simulink model "IEEE34BARRAS"  (R2018a)
settings: Solver=ode4  StartTime=0.0  StopTime=48*T  FixedStep=Ts  RelTol=1e-3  EnableMultiTasking=on
InitFcn:
  | close
  | clc
  | clear
  | n=2^8;
  | f=60;
  | T=1/f;
  | Ts=1/(f*n);
  | NT=18;
  | set_param('IEEE34BARRAS/EMISOR-RECEPTOR/TCP_IP_RX1/ESCRITURA', 'Value','[0,0,0,0,0,0,0,0,0,0,0,0,0,0,0,0,0,0,0,0,0,0,0,0,0,0,0,0,0,0,0,0,0,0,0,0,0,0,0,0,0]')
  | set_param('IEEE34BARRAS/EMISOR-RECEPTOR/TCP_IP_RX1/RETARDO', 'Value','0')
  | run script_client_1_inicio1.m
undefined symbols (not defined in the file or in its folder): D1, Delta, DiscIntNeverNeededParam, Ip1
libraries: powerlib x313, simulink x15, libreria_medidores1 x3, libreria_comunicaciones_cliente1 x2
(part 3 of 5)

== system IEEE34BARRAS/836-862 ==
  Ground : powerlib/Elements/Ground  LConnTagsString=a
  Series RLC Branch1 : powerlib/Elements/Series RLC Branch  LConnTagsString=__new0  RConnTagsString=__new0  BranchType=RL  Resistance=R(1)*Ft  Inductance=L(1)*Ft  SetiL0=off  InitialCurrent=0  Capacitance=8.4659e-09  Setx0=off  InitialVoltage=0  Measurements=None
  Series RLC Branch11 : powerlib/Elements/Series RLC Branch  LConnTagsString=__new0  RConnTagsString=__new0  BranchType=C  Resistance=0.13252  Inductance=0.0024863  SetiL0=off  InitialCurrent=0  Capacitance=C(1)/2*Ft  Setx0=off  InitialVoltage=0  Measurements=None
  Series RLC Branch12 : powerlib/Elements/Series RLC Branch  LConnTagsString=__new0  RConnTagsString=__new0  BranchType=C  Resistance=0.13252  Inductance=0.0024863  SetiL0=off  InitialCurrent=0  Capacitance=C(3)/2*Ft  Setx0=off  InitialVoltage=0  Measurements=None
  Series RLC Branch13 : powerlib/Elements/Series RLC Branch  LConnTagsString=__new0  RConnTagsString=__new0  BranchType=C  Resistance=0.13252  Inductance=0.0024863  SetiL0=off  InitialCurrent=0  Capacitance=C(3)/2*Ft  Setx0=off  InitialVoltage=0  Measurements=None
  Series RLC Branch2 : powerlib/Elements/Series RLC Branch  LConnTagsString=__new0  RConnTagsString=__new0  BranchType=RL  Resistance=R(2)*Ft  Inductance=L(2)*Ft  SetiL0=off  InitialCurrent=0  Capacitance=8.4659e-09  Setx0=off  InitialVoltage=0  Measurements=None
  Series RLC Branch3 : powerlib/Elements/Series RLC Branch  LConnTagsString=__new0  RConnTagsString=__new0  BranchType=C  Resistance=0.13252  Inductance=0.0024863  SetiL0=off  InitialCurrent=0  Capacitance=C(2)/2*Ft  Setx0=off  InitialVoltage=0  Measurements=None
  Series RLC Branch7 : powerlib/Elements/Series RLC Branch  LConnTagsString=__new0  RConnTagsString=__new0  BranchType=C  Resistance=0.13252  Inductance=0.0024863  SetiL0=off  InitialCurrent=0  Capacitance=C(1)/2*Ft  Setx0=off  InitialVoltage=0  Measurements=None
  Series RLC Branch8 : powerlib/Elements/Series RLC Branch  LConnTagsString=__new0  RConnTagsString=__new0  BranchType=C  Resistance=0.13252  Inductance=0.0024863  SetiL0=off  InitialCurrent=0  Capacitance=C(2)/2*Ft  Setx0=off  InitialVoltage=0  Measurements=None
  Series RLC Branch9 : powerlib/Elements/Series RLC Branch  LConnTagsString=__new0  RConnTagsString=__new0  BranchType=RL  Resistance=R(3)*Ft  Inductance=L(3)*Ft  SetiL0=off  InitialCurrent=0  Capacitance=8.4659e-09  Setx0=off  InitialVoltage=0  Measurements=None
  B : PMIOPort  Side=Left
  b : PMIOPort  Port=2  Side=Right
  A : PMIOPort  Port=3  Side=Left
  a : PMIOPort  Port=4  Side=Right
  C : PMIOPort  Port=5  Side=Left
  c : PMIOPort  Port=6  Side=Right
  connections:
  B/RConn1 -- Series RLC Branch11/LConn1 -- Series RLC Branch1/LConn1
  b/RConn1 -- Series RLC Branch7/LConn1 -- Series RLC Branch1/RConn1
  Series RLC Branch8/RConn1 -- Series RLC Branch11/RConn1 -- Series RLC Branch13/RConn1 -- Series RLC Branch12/RConn1 -- Series RLC Branch3/RConn1 -- Series RLC Branch7/RConn1 -- Ground/LConn1
  Series RLC Branch2/LConn1 -- A/RConn1 -- Series RLC Branch8/LConn1
  a/RConn1 -- Series RLC Branch2/RConn1 -- Series RLC Branch3/LConn1
  C/RConn1 -- Series RLC Branch13/LConn1 -- Series RLC Branch9/LConn1
  Series RLC Branch12/LConn1 -- c/RConn1 -- Series RLC Branch9/RConn1

== system IEEE34BARRAS/842-844 ==
  Ground : powerlib/Elements/Ground  LConnTagsString=a
  Series RLC Branch1 : powerlib/Elements/Series RLC Branch  LConnTagsString=__new0  RConnTagsString=__new0  BranchType=RL  Resistance=R(1)*Ft  Inductance=L(1)*Ft  SetiL0=off  InitialCurrent=0  Capacitance=8.4659e-09  Setx0=off  InitialVoltage=0  Measurements=None
  Series RLC Branch11 : powerlib/Elements/Series RLC Branch  LConnTagsString=__new0  RConnTagsString=__new0  BranchType=C  Resistance=0.13252  Inductance=0.0024863  SetiL0=off  InitialCurrent=0  Capacitance=C(1)/2*Ft  Setx0=off  InitialVoltage=0  Measurements=None
  Series RLC Branch12 : powerlib/Elements/Series RLC Branch  LConnTagsString=__new0  RConnTagsString=__new0  BranchType=C  Resistance=0.13252  Inductance=0.0024863  SetiL0=off  InitialCurrent=0  Capacitance=C(3)/2*Ft  Setx0=off  InitialVoltage=0  Measurements=None
  Series RLC Branch13 : powerlib/Elements/Series RLC Branch  LConnTagsString=__new0  RConnTagsString=__new0  BranchType=C  Resistance=0.13252  Inductance=0.0024863  SetiL0=off  InitialCurrent=0  Capacitance=C(3)/2*Ft  Setx0=off  InitialVoltage=0  Measurements=None
  Series RLC Branch2 : powerlib/Elements/Series RLC Branch  LConnTagsString=__new0  RConnTagsString=__new0  BranchType=RL  Resistance=R(2)*Ft  Inductance=L(2)*Ft  SetiL0=off  InitialCurrent=0  Capacitance=8.4659e-09  Setx0=off  InitialVoltage=0  Measurements=None
  Series RLC Branch3 : powerlib/Elements/Series RLC Branch  LConnTagsString=__new0  RConnTagsString=__new0  BranchType=C  Resistance=0.13252  Inductance=0.0024863  SetiL0=off  InitialCurrent=0  Capacitance=C(2)/2*Ft  Setx0=off  InitialVoltage=0  Measurements=None
  Series RLC Branch7 : powerlib/Elements/Series RLC Branch  LConnTagsString=__new0  RConnTagsString=__new0  BranchType=C  Resistance=0.13252  Inductance=0.0024863  SetiL0=off  InitialCurrent=0  Capacitance=C(1)/2*Ft  Setx0=off  InitialVoltage=0  Measurements=None
  Series RLC Branch8 : powerlib/Elements/Series RLC Branch  LConnTagsString=__new0  RConnTagsString=__new0  BranchType=C  Resistance=0.13252  Inductance=0.0024863  SetiL0=off  InitialCurrent=0  Capacitance=C(2)/2*Ft  Setx0=off  InitialVoltage=0  Measurements=None
  Series RLC Branch9 : powerlib/Elements/Series RLC Branch  LConnTagsString=__new0  RConnTagsString=__new0  BranchType=RL  Resistance=R(3)*Ft  Inductance=L(3)*Ft  SetiL0=off  InitialCurrent=0  Capacitance=8.4659e-09  Setx0=off  InitialVoltage=0  Measurements=None
  B : PMIOPort  Side=Left
  b : PMIOPort  Port=2  Side=Right
  A : PMIOPort  Port=3  Side=Left
  a : PMIOPort  Port=4  Side=Right
  C : PMIOPort  Port=5  Side=Left
  c : PMIOPort  Port=6  Side=Right
  connections:
  B/RConn1 -- Series RLC Branch11/LConn1 -- Series RLC Branch1/LConn1
  b/RConn1 -- Series RLC Branch7/LConn1 -- Series RLC Branch1/RConn1
  Series RLC Branch8/RConn1 -- Series RLC Branch11/RConn1 -- Series RLC Branch13/RConn1 -- Series RLC Branch12/RConn1 -- Series RLC Branch3/RConn1 -- Series RLC Branch7/RConn1 -- Ground/LConn1
  Series RLC Branch2/LConn1 -- A/RConn1 -- Series RLC Branch8/LConn1
  a/RConn1 -- Series RLC Branch2/RConn1 -- Series RLC Branch3/LConn1
  C/RConn1 -- Series RLC Branch13/LConn1 -- Series RLC Branch9/LConn1
  Series RLC Branch12/LConn1 -- c/RConn1 -- Series RLC Branch9/RConn1

== system IEEE34BARRAS/844-846 ==
  Ground : powerlib/Elements/Ground  LConnTagsString=a
  Series RLC Branch1 : powerlib/Elements/Series RLC Branch  LConnTagsString=__new0  RConnTagsString=__new0  BranchType=RL  Resistance=R(1)*Ft  Inductance=L(1)*Ft  SetiL0=off  InitialCurrent=0  Capacitance=8.4659e-09  Setx0=off  InitialVoltage=0  Measurements=None
  Series RLC Branch11 : powerlib/Elements/Series RLC Branch  LConnTagsString=__new0  RConnTagsString=__new0  BranchType=C  Resistance=0.13252  Inductance=0.0024863  SetiL0=off  InitialCurrent=0  Capacitance=C(1)/2*Ft  Setx0=off  InitialVoltage=0  Measurements=None
  Series RLC Branch12 : powerlib/Elements/Series RLC Branch  LConnTagsString=__new0  RConnTagsString=__new0  BranchType=C  Resistance=0.13252  Inductance=0.0024863  SetiL0=off  InitialCurrent=0  Capacitance=C(3)/2*Ft  Setx0=off  InitialVoltage=0  Measurements=None
  Series RLC Branch13 : powerlib/Elements/Series RLC Branch  LConnTagsString=__new0  RConnTagsString=__new0  BranchType=C  Resistance=0.13252  Inductance=0.0024863  SetiL0=off  InitialCurrent=0  Capacitance=C(3)/2*Ft  Setx0=off  InitialVoltage=0  Measurements=None
  Series RLC Branch2 : powerlib/Elements/Series RLC Branch  LConnTagsString=__new0  RConnTagsString=__new0  BranchType=RL  Resistance=R(2)*Ft  Inductance=L(2)*Ft  SetiL0=off  InitialCurrent=0  Capacitance=8.4659e-09  Setx0=off  InitialVoltage=0  Measurements=None
  Series RLC Branch3 : powerlib/Elements/Series RLC Branch  LConnTagsString=__new0  RConnTagsString=__new0  BranchType=C  Resistance=0.13252  Inductance=0.0024863  SetiL0=off  InitialCurrent=0  Capacitance=C(2)/2*Ft  Setx0=off  InitialVoltage=0  Measurements=None
  Series RLC Branch7 : powerlib/Elements/Series RLC Branch  LConnTagsString=__new0  RConnTagsString=__new0  BranchType=C  Resistance=0.13252  Inductance=0.0024863  SetiL0=off  InitialCurrent=0  Capacitance=C(1)/2*Ft  Setx0=off  InitialVoltage=0  Measurements=None
  Series RLC Branch8 : powerlib/Elements/Series RLC Branch  LConnTagsString=__new0  RConnTagsString=__new0  BranchType=C  Resistance=0.13252  Inductance=0.0024863  SetiL0=off  InitialCurrent=0  Capacitance=C(2)/2*Ft  Setx0=off  InitialVoltage=0  Measurements=None
  Series RLC Branch9 : powerlib/Elements/Series RLC Branch  LConnTagsString=__new0  RConnTagsString=__new0  BranchType=RL  Resistance=R(3)*Ft  Inductance=L(3)*Ft  SetiL0=off  InitialCurrent=0  Capacitance=8.4659e-09  Setx0=off  InitialVoltage=0  Measurements=None
  B : PMIOPort  Side=Left
  b : PMIOPort  Port=2  Side=Right
  A : PMIOPort  Port=3  Side=Left
  a : PMIOPort  Port=4  Side=Right
  C : PMIOPort  Port=5  Side=Left
  c : PMIOPort  Port=6  Side=Right
  connections:
  c/RConn1 -- Series RLC Branch9/RConn1 -- Series RLC Branch12/LConn1
  C/RConn1 -- Series RLC Branch9/LConn1 -- Series RLC Branch13/LConn1
  a/RConn1 -- Series RLC Branch3/LConn1 -- Series RLC Branch2/RConn1
  A/RConn1 -- Series RLC Branch8/LConn1 -- Series RLC Branch2/LConn1
  Series RLC Branch7/RConn1 -- Series RLC Branch3/RConn1 -- Series RLC Branch13/RConn1 -- Series RLC Branch11/RConn1 -- Series RLC Branch8/RConn1 -- Ground/LConn1 -- Series RLC Branch12/RConn1
  b/RConn1 -- Series RLC Branch1/RConn1 -- Series RLC Branch7/LConn1
  B/RConn1 -- Series RLC Branch1/LConn1 -- Series RLC Branch11/LConn1

== system IEEE34BARRAS/846-848 ==
  Ground : powerlib/Elements/Ground  LConnTagsString=a
  Series RLC Branch1 : powerlib/Elements/Series RLC Branch  LConnTagsString=__new0  RConnTagsString=__new0  BranchType=RL  Resistance=R(1)*Ft  Inductance=L(1)*Ft  SetiL0=off  InitialCurrent=0  Capacitance=8.4659e-09  Setx0=off  InitialVoltage=0  Measurements=None
  Series RLC Branch11 : powerlib/Elements/Series RLC Branch  LConnTagsString=__new0  RConnTagsString=__new0  BranchType=C  Resistance=0.13252  Inductance=0.0024863  SetiL0=off  InitialCurrent=0  Capacitance=C(1)/2*Ft  Setx0=off  InitialVoltage=0  Measurements=None
  Series RLC Branch12 : powerlib/Elements/Series RLC Branch  LConnTagsString=__new0  RConnTagsString=__new0  BranchType=C  Resistance=0.13252  Inductance=0.0024863  SetiL0=off  InitialCurrent=0  Capacitance=C(3)/2*Ft  Setx0=off  InitialVoltage=0  Measurements=None
  Series RLC Branch13 : powerlib/Elements/Series RLC Branch  LConnTagsString=__new0  RConnTagsString=__new0  BranchType=C  Resistance=0.13252  Inductance=0.0024863  SetiL0=off  InitialCurrent=0  Capacitance=C(3)/2*Ft  Setx0=off  InitialVoltage=0  Measurements=None
  Series RLC Branch2 : powerlib/Elements/Series RLC Branch  LConnTagsString=__new0  RConnTagsString=__new0  BranchType=RL  Resistance=R(2)*Ft  Inductance=L(2)*Ft  SetiL0=off  InitialCurrent=0  Capacitance=8.4659e-09  Setx0=off  InitialVoltage=0  Measurements=None
  Series RLC Branch3 : powerlib/Elements/Series RLC Branch  LConnTagsString=__new0  RConnTagsString=__new0  BranchType=C  Resistance=0.13252  Inductance=0.0024863  SetiL0=off  InitialCurrent=0  Capacitance=C(2)/2*Ft  Setx0=off  InitialVoltage=0  Measurements=None
  Series RLC Branch7 : powerlib/Elements/Series RLC Branch  LConnTagsString=__new0  RConnTagsString=__new0  BranchType=C  Resistance=0.13252  Inductance=0.0024863  SetiL0=off  InitialCurrent=0  Capacitance=C(1)/2*Ft  Setx0=off  InitialVoltage=0  Measurements=None
  Series RLC Branch8 : powerlib/Elements/Series RLC Branch  LConnTagsString=__new0  RConnTagsString=__new0  BranchType=C  Resistance=0.13252  Inductance=0.0024863  SetiL0=off  InitialCurrent=0  Capacitance=C(2)/2*Ft  Setx0=off  InitialVoltage=0  Measurements=None
  Series RLC Branch9 : powerlib/Elements/Series RLC Branch  LConnTagsString=__new0  RConnTagsString=__new0  BranchType=RL  Resistance=R(3)*Ft  Inductance=L(3)*Ft  SetiL0=off  InitialCurrent=0  Capacitance=8.4659e-09  Setx0=off  InitialVoltage=0  Measurements=None
  B : PMIOPort  Side=Left
  b : PMIOPort  Port=2  Side=Right
  A : PMIOPort  Port=3  Side=Left
  a : PMIOPort  Port=4  Side=Right
  C : PMIOPort  Port=5  Side=Left
  c : PMIOPort  Port=6  Side=Right
  connections:
  B/RConn1 -- Series RLC Branch11/LConn1 -- Series RLC Branch1/LConn1
  b/RConn1 -- Series RLC Branch7/LConn1 -- Series RLC Branch1/RConn1
  Series RLC Branch8/RConn1 -- Series RLC Branch11/RConn1 -- Series RLC Branch13/RConn1 -- Series RLC Branch12/RConn1 -- Series RLC Branch3/RConn1 -- Series RLC Branch7/RConn1 -- Ground/LConn1
  Series RLC Branch2/LConn1 -- A/RConn1 -- Series RLC Branch8/LConn1
  a/RConn1 -- Series RLC Branch2/RConn1 -- Series RLC Branch3/LConn1
  C/RConn1 -- Series RLC Branch13/LConn1 -- Series RLC Branch9/LConn1
  Series RLC Branch12/LConn1 -- c/RConn1 -- Series RLC Branch9/RConn1

== system IEEE34BARRAS/850-816 ==
  Ground : powerlib/Elements/Ground  LConnTagsString=a
  Series RLC Branch1 : powerlib/Elements/Series RLC Branch  LConnTagsString=__new0  RConnTagsString=__new0  BranchType=RL  Resistance=R(1)*Ft  Inductance=L(1)*Ft  SetiL0=off  InitialCurrent=0  Capacitance=8.4659e-09  Setx0=off  InitialVoltage=0  Measurements=None
  Series RLC Branch11 : powerlib/Elements/Series RLC Branch  LConnTagsString=__new0  RConnTagsString=__new0  BranchType=C  Resistance=0.13252  Inductance=0.0024863  SetiL0=off  InitialCurrent=0  Capacitance=C(1)/2*Ft  Setx0=off  InitialVoltage=0  Measurements=None
  Series RLC Branch12 : powerlib/Elements/Series RLC Branch  LConnTagsString=__new0  RConnTagsString=__new0  BranchType=C  Resistance=0.13252  Inductance=0.0024863  SetiL0=off  InitialCurrent=0  Capacitance=C(3)/2*Ft  Setx0=off  InitialVoltage=0  Measurements=None
  Series RLC Branch13 : powerlib/Elements/Series RLC Branch  LConnTagsString=__new0  RConnTagsString=__new0  BranchType=C  Resistance=0.13252  Inductance=0.0024863  SetiL0=off  InitialCurrent=0  Capacitance=C(3)/2*Ft  Setx0=off  InitialVoltage=0  Measurements=None
  Series RLC Branch2 : powerlib/Elements/Series RLC Branch  LConnTagsString=__new0  RConnTagsString=__new0  BranchType=RL  Resistance=R(2)*Ft  Inductance=L(2)*Ft  SetiL0=off  InitialCurrent=0  Capacitance=8.4659e-09  Setx0=off  InitialVoltage=0  Measurements=None
  Series RLC Branch3 : powerlib/Elements/Series RLC Branch  LConnTagsString=__new0  RConnTagsString=__new0  BranchType=C  Resistance=0.13252  Inductance=0.0024863  SetiL0=off  InitialCurrent=0  Capacitance=C(2)/2*Ft  Setx0=off  InitialVoltage=0  Measurements=None
  Series RLC Branch7 : powerlib/Elements/Series RLC Branch  LConnTagsString=__new0  RConnTagsString=__new0  BranchType=C  Resistance=0.13252  Inductance=0.0024863  SetiL0=off  InitialCurrent=0  Capacitance=C(1)/2*Ft  Setx0=off  InitialVoltage=0  Measurements=None
  Series RLC Branch8 : powerlib/Elements/Series RLC Branch  LConnTagsString=__new0  RConnTagsString=__new0  BranchType=C  Resistance=0.13252  Inductance=0.0024863  SetiL0=off  InitialCurrent=0  Capacitance=C(2)/2*Ft  Setx0=off  InitialVoltage=0  Measurements=None
  Series RLC Branch9 : powerlib/Elements/Series RLC Branch  LConnTagsString=__new0  RConnTagsString=__new0  BranchType=RL  Resistance=R(3)*Ft  Inductance=L(3)*Ft  SetiL0=off  InitialCurrent=0  Capacitance=8.4659e-09  Setx0=off  InitialVoltage=0  Measurements=None
  B : PMIOPort  Side=Left
  b : PMIOPort  Port=2  Side=Right
  A : PMIOPort  Port=3  Side=Left
  a : PMIOPort  Port=4  Side=Right
  C : PMIOPort  Port=5  Side=Left
  c : PMIOPort  Port=6  Side=Right
  connections:
  B/RConn1 -- Series RLC Branch11/LConn1 -- Series RLC Branch1/LConn1
  b/RConn1 -- Series RLC Branch7/LConn1 -- Series RLC Branch1/RConn1
  Series RLC Branch8/RConn1 -- Series RLC Branch11/RConn1 -- Series RLC Branch13/RConn1 -- Series RLC Branch12/RConn1 -- Series RLC Branch3/RConn1 -- Series RLC Branch7/RConn1 -- Ground/LConn1
  Series RLC Branch2/LConn1 -- A/RConn1 -- Series RLC Branch8/LConn1
  a/RConn1 -- Series RLC Branch2/RConn1 -- Series RLC Branch3/LConn1
  C/RConn1 -- Series RLC Branch13/LConn1 -- Series RLC Branch9/LConn1
  Series RLC Branch12/LConn1 -- c/RConn1 -- Series RLC Branch9/RConn1

== system IEEE34BARRAS/852-832 ==
  Ground : powerlib/Elements/Ground  LConnTagsString=a
  Series RLC Branch1 : powerlib/Elements/Series RLC Branch  LConnTagsString=__new0  RConnTagsString=__new0  BranchType=RL  Resistance=R(1)*Ft  Inductance=L(1)*Ft  SetiL0=off  InitialCurrent=0  Capacitance=8.4659e-09  Setx0=off  InitialVoltage=0  Measurements=None
  Series RLC Branch11 : powerlib/Elements/Series RLC Branch  LConnTagsString=__new0  RConnTagsString=__new0  BranchType=C  Resistance=0.13252  Inductance=0.0024863  SetiL0=off  InitialCurrent=0  Capacitance=C(1)/2*Ft  Setx0=off  InitialVoltage=0  Measurements=None
  Series RLC Branch12 : powerlib/Elements/Series RLC Branch  LConnTagsString=__new0  RConnTagsString=__new0  BranchType=C  Resistance=0.13252  Inductance=0.0024863  SetiL0=off  InitialCurrent=0  Capacitance=C(3)/2*Ft  Setx0=off  InitialVoltage=0  Measurements=None
  Series RLC Branch13 : powerlib/Elements/Series RLC Branch  LConnTagsString=__new0  RConnTagsString=__new0  BranchType=C  Resistance=0.13252  Inductance=0.0024863  SetiL0=off  InitialCurrent=0  Capacitance=C(3)/2*Ft  Setx0=off  InitialVoltage=0  Measurements=None
  Series RLC Branch2 : powerlib/Elements/Series RLC Branch  LConnTagsString=__new0  RConnTagsString=__new0  BranchType=RL  Resistance=R(2)*Ft  Inductance=L(2)*Ft  SetiL0=off  InitialCurrent=0  Capacitance=8.4659e-09  Setx0=off  InitialVoltage=0  Measurements=None
  Series RLC Branch3 : powerlib/Elements/Series RLC Branch  LConnTagsString=__new0  RConnTagsString=__new0  BranchType=C  Resistance=0.13252  Inductance=0.0024863  SetiL0=off  InitialCurrent=0  Capacitance=C(2)/2*Ft  Setx0=off  InitialVoltage=0  Measurements=None
  Series RLC Branch7 : powerlib/Elements/Series RLC Branch  LConnTagsString=__new0  RConnTagsString=__new0  BranchType=C  Resistance=0.13252  Inductance=0.0024863  SetiL0=off  InitialCurrent=0  Capacitance=C(1)/2*Ft  Setx0=off  InitialVoltage=0  Measurements=None
  Series RLC Branch8 : powerlib/Elements/Series RLC Branch  LConnTagsString=__new0  RConnTagsString=__new0  BranchType=C  Resistance=0.13252  Inductance=0.0024863  SetiL0=off  InitialCurrent=0  Capacitance=C(2)/2*Ft  Setx0=off  InitialVoltage=0  Measurements=None
  Series RLC Branch9 : powerlib/Elements/Series RLC Branch  LConnTagsString=__new0  RConnTagsString=__new0  BranchType=RL  Resistance=R(3)*Ft  Inductance=L(3)*Ft  SetiL0=off  InitialCurrent=0  Capacitance=8.4659e-09  Setx0=off  InitialVoltage=0  Measurements=None
  B : PMIOPort  Side=Left
  b : PMIOPort  Port=2  Side=Right
  A : PMIOPort  Port=3  Side=Left
  a : PMIOPort  Port=4  Side=Right
  C : PMIOPort  Port=5  Side=Left
  c : PMIOPort  Port=6  Side=Right
  connections:
  B/RConn1 -- Series RLC Branch11/LConn1 -- Series RLC Branch1/LConn1
  b/RConn1 -- Series RLC Branch7/LConn1 -- Series RLC Branch1/RConn1
  Series RLC Branch8/RConn1 -- Series RLC Branch11/RConn1 -- Series RLC Branch13/RConn1 -- Series RLC Branch12/RConn1 -- Series RLC Branch3/RConn1 -- Series RLC Branch7/RConn1 -- Ground/LConn1
  Series RLC Branch2/LConn1 -- A/RConn1 -- Series RLC Branch8/LConn1
  a/RConn1 -- Series RLC Branch2/RConn1 -- Series RLC Branch3/LConn1
  C/RConn1 -- Series RLC Branch13/LConn1 -- Series RLC Branch9/LConn1
  Series RLC Branch12/LConn1 -- c/RConn1 -- Series RLC Branch9/RConn1

== system IEEE34BARRAS/854-852 ==
  Ground : powerlib/Elements/Ground  LConnTagsString=a
  Series RLC Branch1 : powerlib/Elements/Series RLC Branch  LConnTagsString=__new0  RConnTagsString=__new0  BranchType=RL  Resistance=R(1)*Ft  Inductance=L(1)*Ft  SetiL0=off  InitialCurrent=0  Capacitance=8.4659e-09  Setx0=off  InitialVoltage=0  Measurements=None
  Series RLC Branch11 : powerlib/Elements/Series RLC Branch  LConnTagsString=__new0  RConnTagsString=__new0  BranchType=C  Resistance=0.13252  Inductance=0.0024863  SetiL0=off  InitialCurrent=0  Capacitance=C(1)/2*Ft  Setx0=off  InitialVoltage=0  Measurements=None
  Series RLC Branch12 : powerlib/Elements/Series RLC Branch  LConnTagsString=__new0  RConnTagsString=__new0  BranchType=C  Resistance=0.13252  Inductance=0.0024863  SetiL0=off  InitialCurrent=0  Capacitance=C(3)/2*Ft  Setx0=off  InitialVoltage=0  Measurements=None
  Series RLC Branch13 : powerlib/Elements/Series RLC Branch  LConnTagsString=__new0  RConnTagsString=__new0  BranchType=C  Resistance=0.13252  Inductance=0.0024863  SetiL0=off  InitialCurrent=0  Capacitance=C(3)/2*Ft  Setx0=off  InitialVoltage=0  Measurements=None
  Series RLC Branch2 : powerlib/Elements/Series RLC Branch  LConnTagsString=__new0  RConnTagsString=__new0  BranchType=RL  Resistance=R(2)*Ft  Inductance=L(2)*Ft  SetiL0=off  InitialCurrent=0  Capacitance=8.4659e-09  Setx0=off  InitialVoltage=0  Measurements=None
  Series RLC Branch3 : powerlib/Elements/Series RLC Branch  LConnTagsString=__new0  RConnTagsString=__new0  BranchType=C  Resistance=0.13252  Inductance=0.0024863  SetiL0=off  InitialCurrent=0  Capacitance=C(2)/2*Ft  Setx0=off  InitialVoltage=0  Measurements=None
  Series RLC Branch7 : powerlib/Elements/Series RLC Branch  LConnTagsString=__new0  RConnTagsString=__new0  BranchType=C  Resistance=0.13252  Inductance=0.0024863  SetiL0=off  InitialCurrent=0  Capacitance=C(1)/2*Ft  Setx0=off  InitialVoltage=0  Measurements=None
  Series RLC Branch8 : powerlib/Elements/Series RLC Branch  LConnTagsString=__new0  RConnTagsString=__new0  BranchType=C  Resistance=0.13252  Inductance=0.0024863  SetiL0=off  InitialCurrent=0  Capacitance=C(2)/2*Ft  Setx0=off  InitialVoltage=0  Measurements=None
  Series RLC Branch9 : powerlib/Elements/Series RLC Branch  LConnTagsString=__new0  RConnTagsString=__new0  BranchType=RL  Resistance=R(3)*Ft  Inductance=L(3)*Ft  SetiL0=off  InitialCurrent=0  Capacitance=8.4659e-09  Setx0=off  InitialVoltage=0  Measurements=None
  B : PMIOPort  Side=Left
  b : PMIOPort  Port=2  Side=Right
  A : PMIOPort  Port=3  Side=Left
  a : PMIOPort  Port=4  Side=Right
  C : PMIOPort  Port=5  Side=Left
  c : PMIOPort  Port=6  Side=Right
  connections:
  c/RConn1 -- Series RLC Branch9/RConn1 -- Series RLC Branch12/LConn1
  C/RConn1 -- Series RLC Branch9/LConn1 -- Series RLC Branch13/LConn1
  a/RConn1 -- Series RLC Branch3/LConn1 -- Series RLC Branch2/RConn1
  A/RConn1 -- Series RLC Branch8/LConn1 -- Series RLC Branch2/LConn1
  Series RLC Branch7/RConn1 -- Series RLC Branch3/RConn1 -- Series RLC Branch13/RConn1 -- Series RLC Branch11/RConn1 -- Series RLC Branch8/RConn1 -- Ground/LConn1 -- Series RLC Branch12/RConn1
  b/RConn1 -- Series RLC Branch1/RConn1 -- Series RLC Branch7/LConn1
  B/RConn1 -- Series RLC Branch1/LConn1 -- Series RLC Branch11/LConn1

== system IEEE34BARRAS/858-834 ==
  Ground : powerlib/Elements/Ground  LConnTagsString=a
  Series RLC Branch1 : powerlib/Elements/Series RLC Branch  LConnTagsString=__new0  RConnTagsString=__new0  BranchType=RL  Resistance=R(1)*Ft  Inductance=L(1)*Ft  SetiL0=off  InitialCurrent=0  Capacitance=8.4659e-09  Setx0=off  InitialVoltage=0  Measurements=None
  Series RLC Branch11 : powerlib/Elements/Series RLC Branch  LConnTagsString=__new0  RConnTagsString=__new0  BranchType=C  Resistance=0.13252  Inductance=0.0024863  SetiL0=off  InitialCurrent=0  Capacitance=C(1)/2*Ft  Setx0=off  InitialVoltage=0  Measurements=None
  Series RLC Branch12 : powerlib/Elements/Series RLC Branch  LConnTagsString=__new0  RConnTagsString=__new0  BranchType=C  Resistance=0.13252  Inductance=0.0024863  SetiL0=off  InitialCurrent=0  Capacitance=C(3)/2*Ft  Setx0=off  InitialVoltage=0  Measurements=None
  Series RLC Branch13 : powerlib/Elements/Series RLC Branch  LConnTagsString=__new0  RConnTagsString=__new0  BranchType=C  Resistance=0.13252  Inductance=0.0024863  SetiL0=off  InitialCurrent=0  Capacitance=C(3)/2*Ft  Setx0=off  InitialVoltage=0  Measurements=None
  Series RLC Branch2 : powerlib/Elements/Series RLC Branch  LConnTagsString=__new0  RConnTagsString=__new0  BranchType=RL  Resistance=R(2)*Ft  Inductance=L(2)*Ft  SetiL0=off  InitialCurrent=0  Capacitance=8.4659e-09  Setx0=off  InitialVoltage=0  Measurements=None
  Series RLC Branch3 : powerlib/Elements/Series RLC Branch  LConnTagsString=__new0  RConnTagsString=__new0  BranchType=C  Resistance=0.13252  Inductance=0.0024863  SetiL0=off  InitialCurrent=0  Capacitance=C(2)/2*Ft  Setx0=off  InitialVoltage=0  Measurements=None
  Series RLC Branch7 : powerlib/Elements/Series RLC Branch  LConnTagsString=__new0  RConnTagsString=__new0  BranchType=C  Resistance=0.13252  Inductance=0.0024863  SetiL0=off  InitialCurrent=0  Capacitance=C(1)/2*Ft  Setx0=off  InitialVoltage=0  Measurements=None
  Series RLC Branch8 : powerlib/Elements/Series RLC Branch  LConnTagsString=__new0  RConnTagsString=__new0  BranchType=C  Resistance=0.13252  Inductance=0.0024863  SetiL0=off  InitialCurrent=0  Capacitance=C(2)/2*Ft  Setx0=off  InitialVoltage=0  Measurements=None
  Series RLC Branch9 : powerlib/Elements/Series RLC Branch  LConnTagsString=__new0  RConnTagsString=__new0  BranchType=RL  Resistance=R(3)*Ft  Inductance=L(3)*Ft  SetiL0=off  InitialCurrent=0  Capacitance=8.4659e-09  Setx0=off  InitialVoltage=0  Measurements=None
  B : PMIOPort  Side=Left
  b : PMIOPort  Port=2  Side=Right
  A : PMIOPort  Port=3  Side=Left
  a : PMIOPort  Port=4  Side=Right
  C : PMIOPort  Port=5  Side=Left
  c : PMIOPort  Port=6  Side=Right
  connections:
  B/RConn1 -- Series RLC Branch11/LConn1 -- Series RLC Branch1/LConn1
  b/RConn1 -- Series RLC Branch7/LConn1 -- Series RLC Branch1/RConn1
  Series RLC Branch8/RConn1 -- Series RLC Branch11/RConn1 -- Series RLC Branch13/RConn1 -- Series RLC Branch12/RConn1 -- Series RLC Branch3/RConn1 -- Series RLC Branch7/RConn1 -- Ground/LConn1
  Series RLC Branch2/LConn1 -- A/RConn1 -- Series RLC Branch8/LConn1
  a/RConn1 -- Series RLC Branch2/RConn1 -- Series RLC Branch3/LConn1
  C/RConn1 -- Series RLC Branch13/LConn1 -- Series RLC Branch9/LConn1
  Series RLC Branch12/LConn1 -- c/RConn1 -- Series RLC Branch9/RConn1

== system IEEE34BARRAS/860-836 ==
  Ground : powerlib/Elements/Ground  LConnTagsString=a
  Series RLC Branch1 : powerlib/Elements/Series RLC Branch  LConnTagsString=__new0  RConnTagsString=__new0  BranchType=RL  Resistance=R(1)*Ft  Inductance=L(1)*Ft  SetiL0=off  InitialCurrent=0  Capacitance=8.4659e-09  Setx0=off  InitialVoltage=0  Measurements=None
  Series RLC Branch11 : powerlib/Elements/Series RLC Branch  LConnTagsString=__new0  RConnTagsString=__new0  BranchType=C  Resistance=0.13252  Inductance=0.0024863  SetiL0=off  InitialCurrent=0  Capacitance=C(1)/2*Ft  Setx0=off  InitialVoltage=0  Measurements=None
  Series RLC Branch12 : powerlib/Elements/Series RLC Branch  LConnTagsString=__new0  RConnTagsString=__new0  BranchType=C  Resistance=0.13252  Inductance=0.0024863  SetiL0=off  InitialCurrent=0  Capacitance=C(3)/2*Ft  Setx0=off  InitialVoltage=0  Measurements=None
  Series RLC Branch13 : powerlib/Elements/Series RLC Branch  LConnTagsString=__new0  RConnTagsString=__new0  BranchType=C  Resistance=0.13252  Inductance=0.0024863  SetiL0=off  InitialCurrent=0  Capacitance=C(3)/2*Ft  Setx0=off  InitialVoltage=0  Measurements=None
  Series RLC Branch2 : powerlib/Elements/Series RLC Branch  LConnTagsString=__new0  RConnTagsString=__new0  BranchType=RL  Resistance=R(2)*Ft  Inductance=L(2)*Ft  SetiL0=off  InitialCurrent=0  Capacitance=8.4659e-09  Setx0=off  InitialVoltage=0  Measurements=None
  Series RLC Branch3 : powerlib/Elements/Series RLC Branch  LConnTagsString=__new0  RConnTagsString=__new0  BranchType=C  Resistance=0.13252  Inductance=0.0024863  SetiL0=off  InitialCurrent=0  Capacitance=C(2)/2*Ft  Setx0=off  InitialVoltage=0  Measurements=None
  Series RLC Branch7 : powerlib/Elements/Series RLC Branch  LConnTagsString=__new0  RConnTagsString=__new0  BranchType=C  Resistance=0.13252  Inductance=0.0024863  SetiL0=off  InitialCurrent=0  Capacitance=C(1)/2*Ft  Setx0=off  InitialVoltage=0  Measurements=None
  Series RLC Branch8 : powerlib/Elements/Series RLC Branch  LConnTagsString=__new0  RConnTagsString=__new0  BranchType=C  Resistance=0.13252  Inductance=0.0024863  SetiL0=off  InitialCurrent=0  Capacitance=C(2)/2*Ft  Setx0=off  InitialVoltage=0  Measurements=None
  Series RLC Branch9 : powerlib/Elements/Series RLC Branch  LConnTagsString=__new0  RConnTagsString=__new0  BranchType=RL  Resistance=R(3)*Ft  Inductance=L(3)*Ft  SetiL0=off  InitialCurrent=0  Capacitance=8.4659e-09  Setx0=off  InitialVoltage=0  Measurements=None
  B : PMIOPort  Side=Left
  b : PMIOPort  Port=2  Side=Right
  A : PMIOPort  Port=3  Side=Left
  a : PMIOPort  Port=4  Side=Right
  C : PMIOPort  Port=5  Side=Left
  c : PMIOPort  Port=6  Side=Right
  connections:
  c/RConn1 -- Series RLC Branch9/RConn1 -- Series RLC Branch12/LConn1
  C/RConn1 -- Series RLC Branch9/LConn1 -- Series RLC Branch13/LConn1
  a/RConn1 -- Series RLC Branch3/LConn1 -- Series RLC Branch2/RConn1
  A/RConn1 -- Series RLC Branch8/LConn1 -- Series RLC Branch2/LConn1
  Series RLC Branch7/RConn1 -- Series RLC Branch3/RConn1 -- Series RLC Branch13/RConn1 -- Series RLC Branch11/RConn1 -- Series RLC Branch8/RConn1 -- Ground/LConn1 -- Series RLC Branch12/RConn1
  b/RConn1 -- Series RLC Branch1/RConn1 -- Series RLC Branch7/LConn1
  B/RConn1 -- Series RLC Branch1/LConn1 -- Series RLC Branch11/LConn1

== system IEEE34BARRAS/888-890 ==
  Ground : powerlib/Elements/Ground  LConnTagsString=a
  Series RLC Branch1 : powerlib/Elements/Series RLC Branch  LConnTagsString=__new0  RConnTagsString=__new0  BranchType=RL  Resistance=R(1)*Ft  Inductance=L(1)*Ft  SetiL0=off  InitialCurrent=0  Capacitance=8.4659e-09  Setx0=off  InitialVoltage=0  Measurements=None
  Series RLC Branch11 : powerlib/Elements/Series RLC Branch  LConnTagsString=__new0  RConnTagsString=__new0  BranchType=C  Resistance=0.13252  Inductance=0.0024863  SetiL0=off  InitialCurrent=0  Capacitance=C(1)/2*Ft  Setx0=off  InitialVoltage=0  Measurements=None
  Series RLC Branch12 : powerlib/Elements/Series RLC Branch  LConnTagsString=__new0  RConnTagsString=__new0  BranchType=C  Resistance=0.13252  Inductance=0.0024863  SetiL0=off  InitialCurrent=0  Capacitance=C(3)/2*Ft  Setx0=off  InitialVoltage=0  Measurements=None
  Series RLC Branch13 : powerlib/Elements/Series RLC Branch  LConnTagsString=__new0  RConnTagsString=__new0  BranchType=C  Resistance=0.13252  Inductance=0.0024863  SetiL0=off  InitialCurrent=0  Capacitance=C(3)/2*Ft  Setx0=off  InitialVoltage=0  Measurements=None
  Series RLC Branch2 : powerlib/Elements/Series RLC Branch  LConnTagsString=__new0  RConnTagsString=__new0  BranchType=RL  Resistance=R(2)*Ft  Inductance=L(2)*Ft  SetiL0=off  InitialCurrent=0  Capacitance=8.4659e-09  Setx0=off  InitialVoltage=0  Measurements=None
  Series RLC Branch3 : powerlib/Elements/Series RLC Branch  LConnTagsString=__new0  RConnTagsString=__new0  BranchType=C  Resistance=0.13252  Inductance=0.0024863  SetiL0=off  InitialCurrent=0  Capacitance=C(2)/2*Ft  Setx0=off  InitialVoltage=0  Measurements=None
  Series RLC Branch7 : powerlib/Elements/Series RLC Branch  LConnTagsString=__new0  RConnTagsString=__new0  BranchType=C  Resistance=0.13252  Inductance=0.0024863  SetiL0=off  InitialCurrent=0  Capacitance=C(1)/2*Ft  Setx0=off  InitialVoltage=0  Measurements=None
  Series RLC Branch8 : powerlib/Elements/Series RLC Branch  LConnTagsString=__new0  RConnTagsString=__new0  BranchType=C  Resistance=0.13252  Inductance=0.0024863  SetiL0=off  InitialCurrent=0  Capacitance=C(2)/2*Ft  Setx0=off  InitialVoltage=0  Measurements=None
  Series RLC Branch9 : powerlib/Elements/Series RLC Branch  LConnTagsString=__new0  RConnTagsString=__new0  BranchType=RL  Resistance=R(3)*Ft  Inductance=L(3)*Ft  SetiL0=off  InitialCurrent=0  Capacitance=8.4659e-09  Setx0=off  InitialVoltage=0  Measurements=None
  B : PMIOPort  Side=Left
  b : PMIOPort  Port=2  Side=Right
  A : PMIOPort  Port=3  Side=Left
  a : PMIOPort  Port=4  Side=Right
  C : PMIOPort  Port=5  Side=Left
  c : PMIOPort  Port=6  Side=Right
  connections:
  c/RConn1 -- Series RLC Branch9/RConn1 -- Series RLC Branch12/LConn1
  C/RConn1 -- Series RLC Branch9/LConn1 -- Series RLC Branch13/LConn1
  a/RConn1 -- Series RLC Branch3/LConn1 -- Series RLC Branch2/RConn1
  A/RConn1 -- Series RLC Branch8/LConn1 -- Series RLC Branch2/LConn1
  Series RLC Branch7/RConn1 -- Series RLC Branch3/RConn1 -- Series RLC Branch13/RConn1 -- Series RLC Branch11/RConn1 -- Series RLC Branch8/RConn1 -- Ground/LConn1 -- Series RLC Branch12/RConn1
  b/RConn1 -- Series RLC Branch1/RConn1 -- Series RLC Branch7/LConn1
  B/RConn1 -- Series RLC Branch1/LConn1 -- Series RLC Branch11/LConn1

== system IEEE34BARRAS/DL-1 ==
  CD1B : powerlib/Elements/Series RLC Load  LConnTagsString=a  RConnTagsString=__new0  NominalVoltage=14.376e3  NominalFrequency=60  ActivePower=30e3  InductivePower=15e3  CapacitivePower=0  Setx0=off  InitialVoltage=0  SetiL0=off  InitialCurrent=0  Measurements=None  LoadType=constant PQ
  CD1C : powerlib/Elements/Series RLC Load  LConnTagsString=a  RConnTagsString=__new0  NominalVoltage=14.376e3  NominalFrequency=60  ActivePower=25e3  InductivePower=14e3  CapacitivePower=0  Setx0=off  InitialVoltage=0  SetiL0=off  InitialCurrent=0  Measurements=None  LoadType=constant PQ
  Ground13 : powerlib/Elements/Ground  LConnTagsString=a
  Conn1 : PMIOPort  Side=Right
  Conn2 : PMIOPort  Port=2  Side=Right
  connections:
  CD1B/RConn1 -- Conn1/RConn1
  CD1B/LConn1 -- Ground13/LConn1 -- CD1C/LConn1
  CD1C/RConn1 -- Conn2/RConn1

== system IEEE34BARRAS/DL-10 ==
  CD10 : powerlib/Elements/Three-Phase Series RLC Load  LConnTagsString=A|B|C  Configuration=Delta  NominalVoltage=1000  Vabc=[14.376e3,14.376e3,14.376e3]  Vabcp=[24.9e3 24.9e3 24.9e3]  NominalFrequency=60  UnbalancedPower=on  ActivePower=10e3  InductivePower=100  CapacitivePower=0  Pabc=[0 30e3 25e3]  QLabc=[0 15e3 14e3]  QCabc=[0 0 0]  Pabcp=[7e3 2e3 6e3]  QLabcp=[3e3 1e3 3e3]  QCabcp=[0 0 0]  Measurements=None  LoadType=constant Z
  Conn1 : PMIOPort  Side=Left
  Conn2 : PMIOPort  Port=2  Side=Left
  Conn3 : PMIOPort  Port=3  Side=Left
  connections:
  CD10/LConn2 -- Conn2/RConn1
  CD10/LConn3 -- Conn3/RConn1
  CD10/LConn1 -- Conn1/RConn1

== system IEEE34BARRAS/DL-11 ==
  CD11 : powerlib/Elements/Series RLC Load  LConnTagsString=a  RConnTagsString=__new0  NominalVoltage=14.376e3  NominalFrequency=60  ActivePower=2e3  InductivePower=1e3  CapacitivePower=0  Setx0=off  InitialVoltage=0  SetiL0=off  InitialCurrent=0  Measurements=None  LoadType=constant PQ
  Ground7 : powerlib/Elements/Ground  LConnTagsString=a
  Conn1 : PMIOPort  Side=Left
  connections:
  Ground7/LConn1 -- CD11/RConn1
  CD11/LConn1 -- Conn1/RConn1

== system IEEE34BARRAS/DL-12 ==
  CD12 : powerlib/Elements/Three-Phase Series RLC Load  LConnTagsString=A|B|C  Configuration=Delta  NominalVoltage=1000  Vabc=[14.376e3,14.376e3,14.376e3]  Vabcp=[24.9e3 24.9e3 24.9e3]  NominalFrequency=60  UnbalancedPower=on  ActivePower=10e3  InductivePower=100  CapacitivePower=0  Pabc=[0 30e3 25e3]  QLabc=[0 15e3 14e3]  QCabc=[0 0 0]  Pabcp=[4e3 15e3 13e3]  QLabcp=[2e3 8e3 7e3]  QCabcp=[0 0 0]  Measurements=None  LoadType=constant PQ
  Conn1 : PMIOPort  Side=Left
  Conn2 : PMIOPort  Port=2  Side=Left
  Conn3 : PMIOPort  Port=3  Side=Left
  connections:
  CD12/LConn3 -- Conn3/RConn1
  CD12/LConn1 -- Conn1/RConn1
  CD12/LConn2 -- Conn2/RConn1

== system IEEE34BARRAS/DL-13 ==
  CD13 : powerlib/Elements/Three-Phase Series RLC Load  LConnTagsString=A|B|C  Configuration=Delta  NominalVoltage=1000  Vabc=[14.376e3,14.376e3,14.376e3]  Vabcp=[24.9e3 24.9e3 24.9e3]  NominalFrequency=60  UnbalancedPower=on  ActivePower=10e3  InductivePower=100  CapacitivePower=0  Pabc=[0 30e3 25e3]  QLabc=[0 15e3 14e3]  QCabc=[0 0 0]  Pabcp=[16e3 20e3 110e3]  QLabcp=[8e3 10e3 55e3]  QCabcp=[0 0 0]  Measurements=None  LoadType=constant Z
  Conn1 : PMIOPort  Side=Left
  Conn2 : PMIOPort  Port=2  Side=Left
  Conn3 : PMIOPort  Port=3  Side=Left
  connections:
  CD13/LConn3 -- Conn3/RConn1
  CD13/LConn2 -- Conn2/RConn1
  CD13/LConn1 -- Conn1/RConn1

== system IEEE34BARRAS/DL-14 ==
  CD14 : powerlib/Elements/Three-Phase Series RLC Load  LConnTagsString=A|B|C  Configuration=Delta  NominalVoltage=1000  Vabc=[14.376e3,14.376e3,14.376e3]  Vabcp=[24.9e3 24.9e3 24.9e3]  NominalFrequency=60  UnbalancedPower=on  ActivePower=10e3  InductivePower=100  CapacitivePower=0  Pabc=[0 30e3 25e3]  QLabc=[0 15e3 14e3]  QCabc=[0 0 0]  Pabcp=[30e3 10e3 42e3]  QLabcp=[15e3 6e3 22e3]  QCabcp=[0 0 0]  Measurements=None  LoadType=constant PQ
  Conn1 : PMIOPort  Side=Left
  Conn2 : PMIOPort  Port=2  Side=Left
  Conn3 : PMIOPort  Port=3  Side=Left
  connections:
  CD14/LConn2 -- Conn2/RConn1
  CD14/LConn1 -- Conn1/RConn1
  CD14/LConn3 -- Conn3/RConn1

== system IEEE34BARRAS/DL-15 ==
  CD15AB : powerlib/Elements/Series RLC Load  LConnTagsString=a  RConnTagsString=__new0  NominalVoltage=14.376e3  NominalFrequency=60  ActivePower=18e3  InductivePower=9e3  CapacitivePower=0  Setx0=off  InitialVoltage=0  SetiL0=off  InitialCurrent=0  Measurements=None  LoadType=constant I
  CD15BC : powerlib/Elements/Series RLC Load  LConnTagsString=a  RConnTagsString=__new0  NominalVoltage=14.376e3  NominalFrequency=60  ActivePower=22e3  InductivePower=11e3  CapacitivePower=0  Setx0=off  InitialVoltage=0  SetiL0=off  InitialCurrent=0  Measurements=None  LoadType=constant I
  Conn1 : PMIOPort  Side=Right
  Conn2 : PMIOPort  Port=2  Side=Left
  Conn3 : PMIOPort  Port=3  Side=Left
  connections:
  CD15AB/RConn1 -- Conn1/RConn1
  CD15AB/LConn1 -- Conn2/RConn1 -- CD15BC/RConn1
  Conn3/RConn1 -- CD15BC/LConn1

== system IEEE34BARRAS/DL-16 ==
  CD16 : powerlib/Elements/Series RLC Load  LConnTagsString=a  RConnTagsString=__new0  NominalVoltage=14.376e3  NominalFrequency=60  ActivePower=28e3  InductivePower=14e3  CapacitivePower=0  Setx0=off  InitialVoltage=0  SetiL0=off  InitialCurrent=0  Measurements=None  LoadType=constant PQ
  Ground8 : powerlib/Elements/Ground  LConnTagsString=a
  Conn1 : PMIOPort  Side=Left
  connections:
  Ground8/LConn1 -- CD16/RConn1
  Conn1/RConn1 -- CD16/LConn1

== system IEEE34BARRAS/DL-17 ==
  CD17 : powerlib/Elements/Series RLC Load  LConnTagsString=a  RConnTagsString=__new0  NominalVoltage=14.376e3  NominalFrequency=60  ActivePower=9e3  InductivePower=5e3  CapacitivePower=0  Setx0=off  InitialVoltage=0  SetiL0=off  InitialCurrent=0  Measurements=None  LoadType=constant PQ
  Ground9 : powerlib/Elements/Ground  LConnTagsString=a
  Conn1 : PMIOPort  Side=Left
  connections:
  Ground9/LConn1 -- CD17/RConn1
  CD17/LConn1 -- Conn1/RConn1

== system IEEE34BARRAS/DL-18 ==
  CD18B : powerlib/Elements/Series RLC Load  LConnTagsString=a  RConnTagsString=__new0  NominalVoltage=14.376e3  NominalFrequency=60  ActivePower=25e3  InductivePower=20e3  CapacitivePower=0  Setx0=off  InitialVoltage=0  SetiL0=off  InitialCurrent=0  Measurements=None  LoadType=constant I
  CD18C : powerlib/Elements/Series RLC Load  LConnTagsString=a  RConnTagsString=__new0  NominalVoltage=14.376e3  NominalFrequency=60  ActivePower=20e3  InductivePower=11e3  CapacitivePower=0  Setx0=off  InitialVoltage=0  SetiL0=off  InitialCurrent=0  Measurements=None  LoadType=constant I
  Ground14 : powerlib/Elements/Ground  LConnTagsString=a
  Conn1 : PMIOPort  Side=Right
  Conn2 : PMIOPort  Port=2  Side=Right
  connections:
  CD18C/LConn1 -- Ground14/LConn1 -- CD18B/LConn1
  Conn2/RConn1 -- CD18C/RConn1
  CD18B/RConn1 -- Conn1/RConn1

== system IEEE34BARRAS/DL-19 ==
  CD19 : powerlib/Elements/Series RLC Load  LConnTagsString=a  RConnTagsString=__new0  NominalVoltage=14.376e3  NominalFrequency=60  ActivePower=23e3  InductivePower=11e3  CapacitivePower=0  Setx0=off  InitialVoltage=0  SetiL0=off  InitialCurrent=0  Measurements=None  LoadType=constant PQ
  Ground10 : powerlib/Elements/Ground  LConnTagsString=a
  Conn1 : PMIOPort  Side=Left
  connections:
  CD19/LConn1 -- Conn1/RConn1
  Ground10/LConn1 -- CD19/RConn1

== system IEEE34BARRAS/DL-2 ==
  CD02 : powerlib/Elements/Series RLC Load  LConnTagsString=a  RConnTagsString=__new0  NominalVoltage=14.376e3  NominalFrequency=60  ActivePower=16e3  InductivePower=8e3  CapacitivePower=0  Setx0=off  InitialVoltage=0  SetiL0=off  InitialCurrent=0  Measurements=None  LoadType=constant I
  Ground : powerlib/Elements/Ground  LConnTagsString=a
  Conn1 : PMIOPort  Side=Left
  connections:
  Ground/LConn1 -- CD02/RConn1
  CD02/LConn1 -- Conn1/RConn1

== system IEEE34BARRAS/DL-3 ==
  CD03 : powerlib/Elements/Series RLC Load  LConnTagsString=a  RConnTagsString=__new0  NominalVoltage=14.376e3  NominalFrequency=60  ActivePower=34e3  InductivePower=17e3  CapacitivePower=0  Setx0=off  InitialVoltage=0  SetiL0=off  InitialCurrent=0  Measurements=None  LoadType=constant Z
  Ground1 : powerlib/Elements/Ground  LConnTagsString=a
  Conn1 : PMIOPort  Side=Left
  connections:
  Ground1/LConn1 -- CD03/RConn1
  CD03/LConn1 -- Conn1/RConn1

== system IEEE34BARRAS/DL-4 ==
  CD04 : powerlib/Elements/Series RLC Load  LConnTagsString=a  RConnTagsString=__new0  NominalVoltage=14.376e3  NominalFrequency=60  ActivePower=135e3  InductivePower=70e3  CapacitivePower=0  Setx0=off  InitialVoltage=0  SetiL0=off  InitialCurrent=0  Measurements=None  LoadType=constant PQ
  Ground2 : powerlib/Elements/Ground  LConnTagsString=a
  Conn1 : PMIOPort  Side=Left
  connections:
  Ground2/LConn1 -- CD04/RConn1
  CD04/LConn1 -- Conn1/RConn1

== system IEEE34BARRAS/DL-5 ==
  CD05 : powerlib/Elements/Series RLC Load  LConnTagsString=a  RConnTagsString=__new0  NominalVoltage=24.9e3  NominalFrequency=60  ActivePower=5e3  InductivePower=2e3  CapacitivePower=0  Setx0=off  InitialVoltage=0  SetiL0=off  InitialCurrent=0  Measurements=None  LoadType=constant I
  Conn1 : PMIOPort  Side=Left
  Conn2 : PMIOPort  Port=2  Side=Right
  connections:
  CD05/RConn1 -- Conn2/RConn1
  CD05/LConn1 -- Conn1/RConn1

== system IEEE34BARRAS/DL-6 ==
  CD06 : powerlib/Elements/Series RLC Load  LConnTagsString=a  RConnTagsString=__new0  NominalVoltage=14.376e3  NominalFrequency=60  ActivePower=40e3  InductivePower=20e3  CapacitivePower=0  Setx0=off  InitialVoltage=0  SetiL0=off  InitialCurrent=0  Measurements=None  LoadType=constant I
  Ground3 : powerlib/Elements/Ground  LConnTagsString=a
  Conn1 : PMIOPort  Side=Left
  connections:
  Ground3/LConn1 -- CD06/RConn1
  CD06/LConn1 -- Conn1/RConn1

== system IEEE34BARRAS/DL-7 ==
  CD07 : powerlib/Elements/Series RLC Load  LConnTagsString=a  RConnTagsString=__new0  NominalVoltage=14.376e3  NominalFrequency=60  ActivePower=4e3  InductivePower=2e3  CapacitivePower=0  Setx0=off  InitialVoltage=0  SetiL0=off  InitialCurrent=0  Measurements=None  LoadType=constant PQ
  Ground4 : powerlib/Elements/Ground  LConnTagsString=a
  Conn1 : PMIOPort  Side=Left
  connections:
  Ground4/LConn1 -- CD07/RConn1
  CD07/LConn1 -- Conn1/RConn1

== system IEEE34BARRAS/DL-8 ==
  CD08 : powerlib/Elements/Series RLC Load  LConnTagsString=a  RConnTagsString=__new0  NominalVoltage=14.376e3  NominalFrequency=60  ActivePower=7e3  InductivePower=3e3  CapacitivePower=0  Setx0=off  InitialVoltage=0  SetiL0=off  InitialCurrent=0  Measurements=None  LoadType=constant PQ
  Ground6 : powerlib/Elements/Ground  LConnTagsString=a
  Conn1 : PMIOPort  Side=Left
  connections:
  Ground6/LConn1 -- CD08/RConn1
  CD08/LConn1 -- Conn1/RConn1

== system IEEE34BARRAS/DL-9 ==
  CD09 : powerlib/Elements/Series RLC Load  LConnTagsString=a  RConnTagsString=__new0  NominalVoltage=14.376e3  NominalFrequency=60  ActivePower=4e3  InductivePower=2e3  CapacitivePower=0  Setx0=off  InitialVoltage=0  SetiL0=off  InitialCurrent=0  Measurements=None  LoadType=constant PQ
  Ground5 : powerlib/Elements/Ground  LConnTagsString=a
  Conn1 : PMIOPort  Side=Left
  connections:
  Ground5/LConn1 -- CD09/RConn1
  Conn1/RConn1 -- CD09/LConn1

== system IEEE34BARRAS/EMISOR-RECEPTOR ==
  note: Transmisión de datos
  note: Recepción de datos
  In1 : Inport
  In2 : Inport  Port=2
  In3 : Inport  Port=3
  Display1 : Display
  Mux : Mux  Inputs=3
  TCP_IP_RX1 : libreria_comunicaciones_cliente1/TCP_IP_RX1  SystemSampleTime=-1
      link override ESCRITURA: Value=client_1.dato_lectura
      link override RETARDO: Value=e
      settings: SourceProductName=The database C:\Users\ana-n\AppData\Roaming\MathWorks\MATLAB\R2018a\slblocks_master.db is locked, or a table in the database is locked. (database is locked)
  TCP_IP_TX1 : libreria_comunicaciones_cliente1/TCP_IP_TX1  SystemSampleTime=-1
      settings: SourceProductName=The database C:\Users\ana-n\AppData\Roaming\MathWorks\MATLAB\R2018a\slblocks_master.db is locked, or a table in the database is locked. (database is locked)
  Out1 : Outport
  Out2 : Outport  Port=2
  Out3 : Outport  Port=3
  Out4 : Outport  Port=4
  Out5 : Outport  Port=5
  Out6 : Outport  Port=6
  Out7 : Outport  Port=7
  Out8 : Outport  Port=8
  wires:
  TCP_IP_RX1/1 -> Out8/1
  TCP_IP_RX1/7 -> Out2/1
  TCP_IP_RX1/5 -> Out4/1
  TCP_IP_RX1/3 -> Out6/1
  Mux/1 -> TCP_IP_TX1/1, Display1/1
  TCP_IP_RX1/4 -> Out5/1
  TCP_IP_RX1/2 -> Out7/1
  TCP_IP_RX1/8 -> Out1/1
  TCP_IP_RX1/6 -> Out3/1
  In3/1 -> Mux/3
  In2/1 -> Mux/2
  In1/1 -> Mux/1

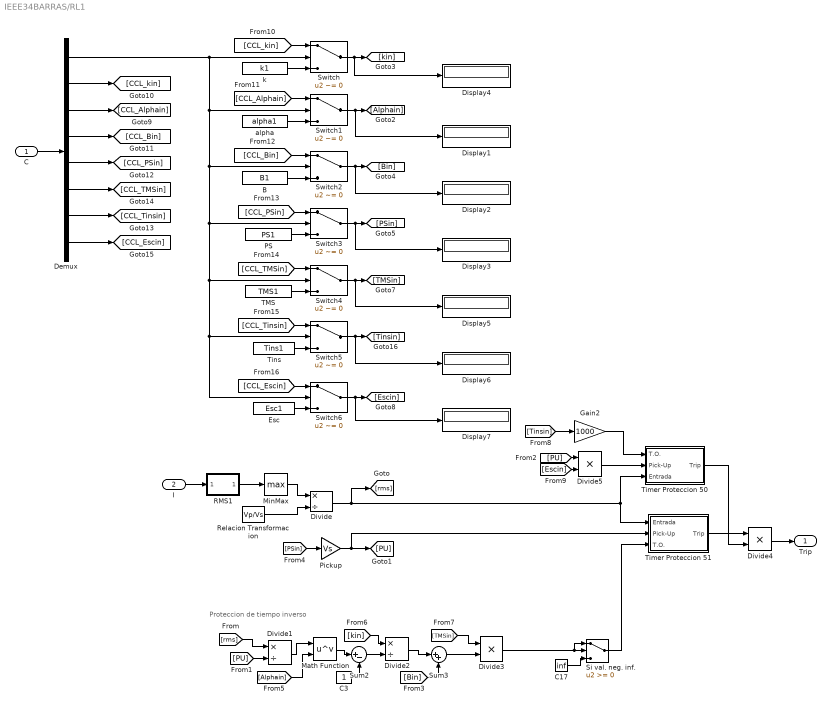
== system IEEE34BARRAS/RL1 ==
  note: Proteccion de tiempo inverso
  C : Inport
  I : Inport  Port=2
  B : Constant  Value=B1
  C17 : Constant  Value=inf
  C3 : Constant
  Demux : Demux  Outputs=8
  Display{1..7} (7 alike) : Display
  Divide : Product  Inputs=*/
  Divide1 : Product  Inputs=*/
  Divide2 : Product  Inputs=*/
  Divide3 : Product  Inputs=**
  Divide4 : Product  Inputs=**
  Divide5 : Product  Inputs=**
  Esc : Constant  Value=Esc1
  Gain2 : Gain  Gain=1000
  Math Function : Math  Operator=pow  SaturateOnIntegerOverflow=on
  MinMax : MinMax  Function=max
  PS : Constant  Value=PS1
  Pickup : Gain  Gain=Vs
  RMS1 : Subsystem
  Relacion Transformacion : Constant  Value=Vp/Vs
  Si val. neg. inf. : Switch
  Sum2 : Sum  Inputs=|+-
  Sum3 : Sum  Inputs=|++
  Switch{,1..6} (7 alike) : Switch  Criteria=u2 ~= 0
  TMS : Constant  Value=TMS1
  Timer Proteccion 50 : Subsystem
  Timer Proteccion 51 : Subsystem
  Tins : Constant  Value=Tins1
  alpha : Constant  Value=alpha1
  k : Constant  Value=k1
  Trip : Outport
  wires:
  Divide4/1 -> Trip/1
  [Escin] -> Divide5/2
  C17/1 -> Si val. neg. inf./3
  Math Function/1 -> Sum2/1
  [kin] -> Divide2/1
  Timer Proteccion 50/1(Trip) -> Divide4/2
  [PSin] -> Pickup/1
  Si val. neg. inf./1 -> Timer Proteccion 51/3(T.O.)
  [Tinsin] -> Gain2/1
  Timer Proteccion 51/1(Trip) -> Divide4/1
  [Alphain] -> Math Function/2
  [PU] -> Divide1/2
  [PU] -> Divide5/1
  Divide5/1 -> Timer Proteccion 50/2(Pick-Up)
  Divide2/1 -> Sum3/1
  Gain2/1 -> Timer Proteccion 50/1(T.O.)
  Divide3/1 -> Si val. neg. inf./1, Si val. neg. inf./2
  Sum3/1 -> Divide3/2
  [Bin] -> Sum3/2
  Relacion Transformacion/1 -> Divide/2
  Divide/1 -> Timer Proteccion 50/3(Entrada), Timer Proteccion 51/1(Entrada), [rms]
  Sum2/1 -> Divide2/2
  Divide1/1 -> Math Function/1
  [rms] -> Divide1/1
  Pickup/1 -> Timer Proteccion 51/2(Pick-Up), [PU]
  MinMax/1 -> Divide/1
  RMS1/1(Out1) -> MinMax/1
  [TMSin] -> Divide3/1
  C3/1 -> Sum2/2
  I/1 -> RMS1/1(In1)
  C/1 -> Demux/1
  Demux/1 -> Switch2/2, Switch4/2, Switch6/2, Switch5/2, Switch3/2, Switch1/2, Switch/2
  Demux/7 -> [CCL_Tinsin]
  Demux/5 -> [CCL_PSin]
  Demux/4 -> [CCL_Bin]
  Demux/2 -> [CCL_kin]
  Demux/3 -> [CCL_Alphain]
  Demux/6 -> [CCL_TMSin]
  Demux/8 -> [CCL_Escin]
  B/1 -> Switch2/3
  PS/1 -> Switch3/3
  TMS/1 -> Switch4/3
  Tins/1 -> Switch5/3
  Esc/1 -> Switch6/3
  Switch/1 -> Display4/1, [kin]
  Switch1/1 -> Display1/1, [Alphain]
  Switch3/1 -> Display3/1, [PSin]
  Switch4/1 -> Display5/1, [TMSin]
  Switch5/1 -> Display6/1, [Tinsin]
  Switch6/1 -> Display7/1, [Escin]
  alpha/1 -> Switch1/3
  [CCL_Alphain] -> Switch1/1
  [CCL_Bin] -> Switch2/1
  [CCL_PSin] -> Switch3/1
  [CCL_TMSin] -> Switch4/1
  [CCL_Tinsin] -> Switch5/1
  [CCL_Escin] -> Switch6/1
  k/1 -> Switch/3
  [CCL_kin] -> Switch/1
  Switch2/1 -> Display2/1, [Bin]
